simulink model "KalmanBoucleModel"  (Simulink 7.4)
settings: Solver=ode45  StartTime=0.0  StopTime=10.0  RelTol=1e-3
values from neighbouring files (symbols this model uses):
  Mesure = zeros(8,N)    [Kalman_routine.m]    (also in Kalman_routine2.m)
  P0 = eye(2)    [Kalman_routine.m]    (also in Kalman_routine2.m)
  R = [Rgps     0       0       0       0       0       0       0 ... (first row only)    [Kalman_routine.m]    (also in Kalman_routine2.m)
  X0 = zeros(2,1)    [Kalman_routine.m]    (also in Kalman_routine2.m)
  Z0 = zeros(8,1)    [Kalman_routine.m]    (also in Kalman_routine2.m)
settings Model: Creator=Dim_Compaq  LastModifiedBy=Dim_Compaq

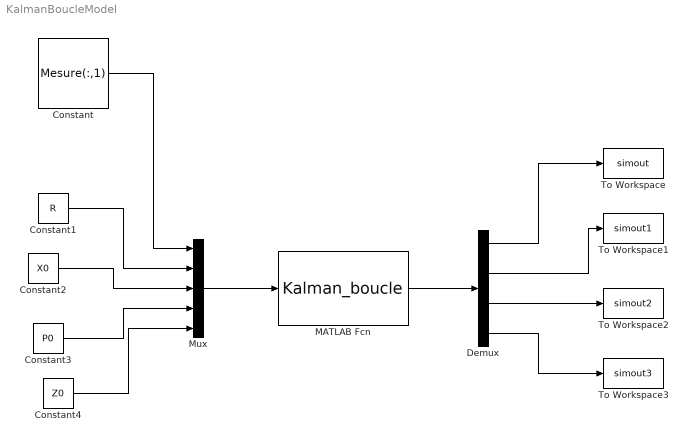
== system KalmanBoucleModel ==
  Constant : Constant  Value=Mesure(:,1)  OutDataType=fixdt(1, 16)  OutScaling=2^0
  Constant1 : Constant  Value=R  OutDataType=fixdt(1, 16)  OutScaling=2^0
  Constant2 : Constant  Value=X0  OutDataType=fixdt(1, 16)  OutScaling=2^0
  Constant3 : Constant  Value=P0  OutDataType=fixdt(1, 16)  OutScaling=2^0
  Constant4 : Constant  Value=Z0  OutDataType=fixdt(1, 16)  OutScaling=2^0
  Demux : Demux
  MATLAB Fcn : MATLABFcn  MATLABFcn=Kalman_boucle
  Mux : Mux  Inputs=5
  To Workspace : ToWorkspace  VariableName=simout  SampleTime=-1  SaveFormat=Structure
  To Workspace1 : ToWorkspace  VariableName=simout1  SampleTime=-1  SaveFormat=Structure
  To Workspace2 : ToWorkspace  VariableName=simout2  SampleTime=-1  SaveFormat=Structure
  To Workspace3 : ToWorkspace  VariableName=simout3  SampleTime=-1  SaveFormat=Structure
  wires:
  Mux/1 -> MATLAB Fcn/1
  MATLAB Fcn/1 -> Demux/1
  Constant/1 -> Mux/1
  Constant1/1 -> Mux/2
  Constant2/1 -> Mux/3
  Constant3/1 -> Mux/4
  Constant4/1 -> Mux/5
  Demux/1 -> To Workspace/1
  Demux/2 -> To Workspace1/1
  Demux/3 -> To Workspace2/1
  Demux/4 -> To Workspace3/1
